simulink model "week1problem1"  (R2020a)
settings: Solver=VariableStepAuto  StartTime=0.0  StopTime=10  MaxStep=0.01  RelTol=1e-3
values from neighbouring files (symbols this model uses):
  b = 50    [week1problem1.mat]
  K1 = 50    [week1problem1.mat]
  K12 = 10002    [week1problem1.mat]
  M1 = 100    [week1problem1.mat]
  M2 = 104    [week1problem1.mat]
settings Model: Creator=Admin  LastModifiedBy=Admin

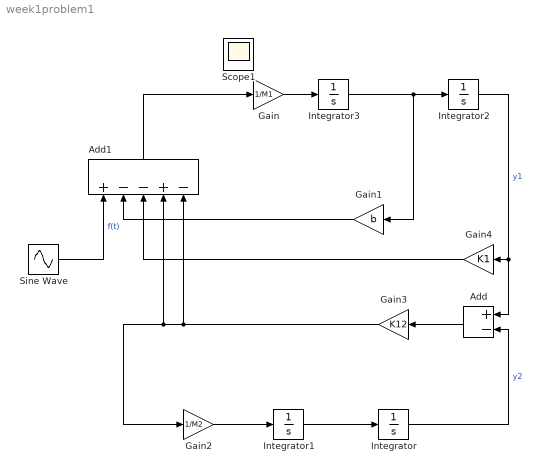
== system week1problem1 ==
  Add : Sum  Inputs=+-
  Add1 : Sum  Inputs=+--+-
  Gain : Gain  Gain=1/M1
  Gain1 : Gain  Gain=b
  Gain2 : Gain  Gain=1/M2
  Gain3 : Gain  Gain=K12
  Gain4 : Gain  Gain=K1
  Integrator{,1..3} (4 alike) : Integrator
  Sine Wave : Sin  Amplitude=2  Frequency=2*pi*10  SampleTime=0
  Scope1 : Scope
  wires:
  Add1/1 -> Gain/1
  Integrator3/1 -> Gain1/1, Integrator2/1
  Gain1/1 -> Add1/2
  Gain4/1 -> Add1/3
  Integrator2/1 -> Add/1, Gain4/1  "y1"
  Add/1 -> Gain3/1
  Gain3/1 -> Add1/5, Gain2/1, Add1/4
  Gain2/1 -> Integrator1/1
  Integrator1/1 -> Integrator/1
  Integrator/1 -> Add/2  "y2"
  Sine Wave/1 -> Add1/1  "f(t)"
  Gain/1 -> Integrator3/1
